simulink model "WDGBrakeTimeCalc_Harness"  (R2024a)
settings: configuration reference "csMultiInstance" (kept outside this file)
settings Model: DataDictionary=DD_WDGBrakeTimeCalc.sldd  Creator=The MathWorks, Inc.  LastModifiedBy=The MathWorks, Inc.
settings ConfigSetRef: SourceName=csMultiInstance

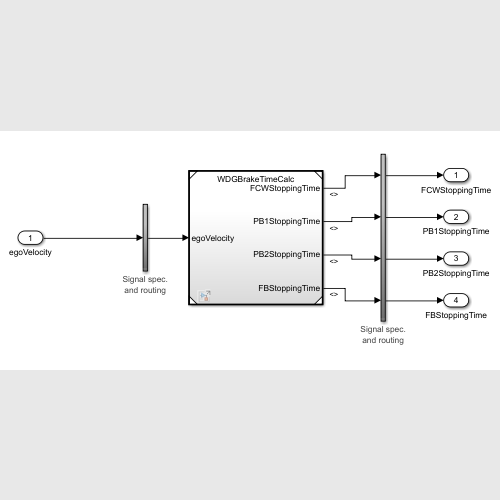
[thumbnail: Simulink's stored preview of the top-level diagram]
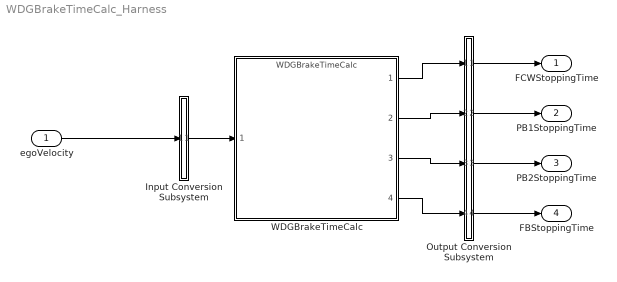
== system WDGBrakeTimeCalc_Harness ==
  egoVelocity : Inport  OutDataTypeStr=double  PortDimensions=[1]  SampleTime=0.1
  Input Conversion Subsystem : Subsystem  Tag=__SLT_ICS__  Description=|
      | Signal spec.
      | and routing
      settings: AttributesFormatString=%<Description>
  Output Conversion Subsystem : Subsystem  Tag=__SLT_OCS__  Description=|
      | Signal spec.
      | and routing
      settings: AttributesFormatString=%<Description>
  WDGBrakeTimeCalc : ModelReference  ModelNameDialog=WDGBrakeTimeCalc  SimulationMode=Normal  ModelReferenceVersion=7.0
  FCWStoppingTime : Outport
  PB1StoppingTime : Outport  Port=2
  PB2StoppingTime : Outport  Port=3
  FBStoppingTime : Outport  Port=4
  wires:
  egoVelocity/1 -> Input Conversion Subsystem/1(Inport_1)
  Output Conversion Subsystem/1(Outport_1) -> FCWStoppingTime/1
  Output Conversion Subsystem/2(Outport_2) -> PB1StoppingTime/1
  Output Conversion Subsystem/3(Outport_3) -> PB2StoppingTime/1
  Output Conversion Subsystem/4(Outport_4) -> FBStoppingTime/1
  Input Conversion Subsystem/1(Outport_1) -> WDGBrakeTimeCalc/1
  WDGBrakeTimeCalc/1 -> Output Conversion Subsystem/1(Inport_1)
  WDGBrakeTimeCalc/2 -> Output Conversion Subsystem/2(Inport_2)
  WDGBrakeTimeCalc/3 -> Output Conversion Subsystem/3(Inport_3)
  WDGBrakeTimeCalc/4 -> Output Conversion Subsystem/4(Inport_4)

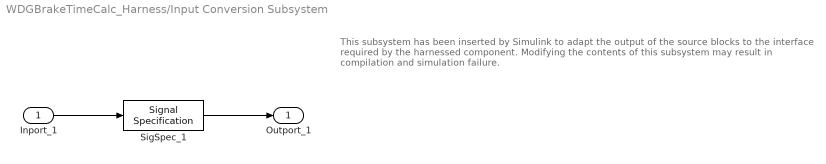
== system WDGBrakeTimeCalc_Harness/Input Conversion Subsystem ==
  note: This subsystem has been inserted by Simulink to adapt the output of the source blocks to the interface required by the harnessed component.
      |  Modifying the contents of this subsystem may result in compilation and simulation failure.
  Inport_1 : Inport
  SigSpec_1 : SignalSpecification  OutDataTypeStr=double  Unit=m/s  Dimensions=[1]  SampleTime=0.1
  Outport_1 : Outport
  wires:
  SigSpec_1/1 -> Outport_1/1
  Inport_1/1 -> SigSpec_1/1

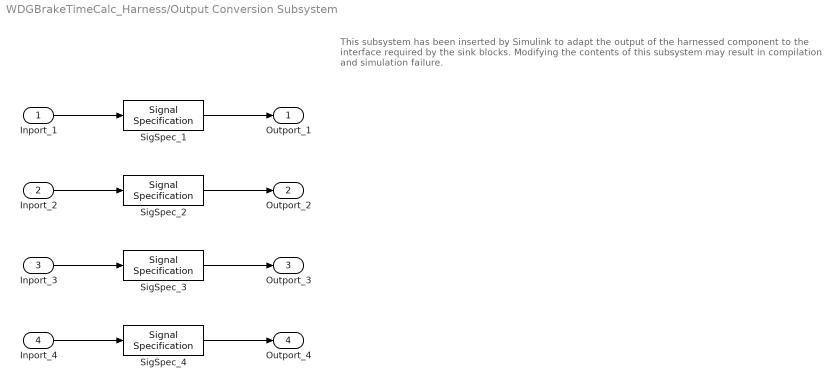
== system WDGBrakeTimeCalc_Harness/Output Conversion Subsystem ==
  note: This subsystem has been inserted by Simulink to adapt the output of the harnessed component to the interface required by the sink blocks.
      |  Modifying the contents of this subsystem may result in compilation and simulation failure.
  Inport_1 : Inport
  Inport_2 : Inport  Port=2
  Inport_3 : Inport  Port=3
  Inport_4 : Inport  Port=4
  SigSpec_{1..4} (4 alike) : SignalSpecification  OutDataTypeStr=double  Unit=s  Dimensions=[1]  SampleTime=0.1
  Outport_1 : Outport
  Outport_2 : Outport  Port=2
  Outport_3 : Outport  Port=3
  Outport_4 : Outport  Port=4
  wires:
  Inport_1/1 -> SigSpec_1/1
  SigSpec_1/1 -> Outport_1/1
  Inport_2/1 -> SigSpec_2/1
  SigSpec_2/1 -> Outport_2/1
  Inport_3/1 -> SigSpec_3/1
  SigSpec_3/1 -> Outport_3/1
  Inport_4/1 -> SigSpec_4/1
  SigSpec_4/1 -> Outport_4/1
